simulink model "narx"  (R2019a)
settings: Solver=VariableStepAuto  StartTime=0.0  StopTime=10.0  RelTol=1e-3
libraries: neural x208
(part 2 of 4)

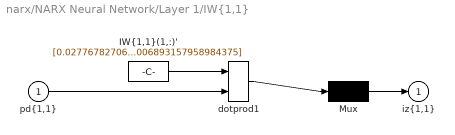
== system narx/NARX Neural Network/Layer 1/IW{1,1} ==
  "pd{1,1}" : Inport  PortDimensions=400  SampleTime=0.1
      mask Display: e = 0.06;c1 = [120 230 180]/255;c2 = ([120 230 180]+0)/(256+128);c3 = ([120 230 180]+128)/(256+128);patch([0 1 1 0],[0 0 1 1],c1);patch([0 1 1 1-e 1-e 0+e],[0 0 1 1-e 0+e 0+e],c2);patch([0 0 1 1-e 0+e 0+e],[0 1 1 1-e 1-e 0+e],c3);plot([0 1 1 0 0],[0 0 1 1 0]);
  "IW{1,1}(1,:)'" : Constant  Value=[0.0277678270648271420528718778086840757168829441070556640625;-0.072495516445331864563428325709537602961063385009765625;0.0729014756815358488939438075249199755489826202392578125;-0.07750431119418264847009680806877440772950649261474609375;0.08403681875376804721877732617940637283027172088623046875;0.034610402156992348121633540358743630349636077880859375;0.062177287459774917277588457409365219064056873321533203125;-0.055599584925755320130580372506301500834524631500244140625;0.03306038363780137989689222877132124267518520355224609375;0.059884523458899295567103848725309944711625576019287109375;-0.045214944417939294252217763414591900072991847991943359375;-0.06297951265383126828734106084084487520158290863037109375;-0.07549611905665236377682703050595591776072978973388671875;0.0244025606892776560086222303880276740528643131256103515625;-0.07090652620408342821090030838604434393346309661865234375;0.046678136882927552531175052763501298613846302032470703125;0.01041356304968433198199218026047674356959760189056396484375;-0.0682147965948884105191751814345479942858219146728515625;0.0395052435226136144930109139750129543244838714599609375;-0.01285278232501787902541945385337385232560336589813232421875;0.0297225523606888426819683246549175237305462360382080078125;0.052786377986352495117472471974906511604785919189453125;0.06689768777292716406268624496078700758516788482666015625;0.029275876104348765027740597588490345515310764312744140625;0.056569434444663994898672143563089775852859020233154296875;0.0801803794504956091060421385918743908405303955078125;0.04308993957098707083819277841030270792543888092041015625;0.01449172193578054414209166367299985722638666629791259765625;0.07754270635757322394088220107732922770082950592041015625;-0.04770856845629760367710758828252437524497509002685546875;-0.049209625536573896320557963690589531324803829193115234375;0.0831284199689841518665645025976118631660938262939453125;0.0035056066225432809015105650729537956067360937595367431640625;-0.0437420353957994889615434885854483582079410552978515625;-0.018606367207281183928646584035959676839411258697509765625;-0.04804876946083826150246665065424167551100254058837890625;-0.03351981478313360851561952813426614739000797271728515625;0.032643606251778249649486696171152289025485515594482421875;0.021534071288703326985114472336135804653167724609375;-0.06660372496869400305019581765009206719696521759033203125;-0.035615956814750070191788466900106868706643581390380859375;0.0179231172393173980583735982463622349314391613006591796875;0.06328180682564453485294819756745710037648677825927734375;0.054315872080360309837043786274080048315227031707763671875;-0.02052611847061401595393448360482580028474330902099609375;-0.0021784938142405513815391682186373145668767392635345458984375;0.0478869794394115866342787057874375022947788238525390625;-0.047002427956548124832192314670464838854968547821044921875;-0.0578385735760633679092279635369777679443359375;-0.042262951181773596165403006352789816446602344512939453125;0.08173333373884129893216510254205786623060703277587890625;0.007633612464141942451079092535337622393853962421417236328125;0.0286695925062813126993344070569946779869496822357177734375;0.0301009651872837340202959666157767060212790966033935546875;0.0200074381308329267425971664806638727895915508270263671875;-0.0728720042760638564427466690176515839993953704833984375;-0.005924178409521227255118969168279363657347857952117919921875;-0.02458613042365609402395421057008206844329833984375;0.018579335229139327945180326651097857393324375152587890625;0.0197572222726313286023103188426830456592142581939697265625;-0.03253055515353310556125876473743119277060031890869140625;0.058288896225512872029117517058693920262157917022705078125;-0.054834929476499406908462930232417420484125614166259765625;-0.083249590273886397984171026109834201633930206298828125;-0.04734203805234958595260508218416362069547176361083984375;0.006637613387688349846083024630161162349395453929901123046875 ...(+20044 chars)]
      mask Display: e = 0.06;c1 = [120 150 230]/255;c2 = ([120 150 230]+0)/383;c3 = ([120 150 230]+128)/383;patch([0 1 1 0],[0 0 1 1],c1);patch([0 1 1 1-e 1-e 0+e],[0 0 1 1-e 0+e 0+e],c2);patch([0 0 1 1-e 0+e 0+e],[0 1 1 1-e 1-e 0+e],c3);plot([0 1 1 0 0],[0 0 1 1 0]);disp('Weights');
  Mux : Mux  Inputs=1
      mask Display: e = 0.06;c1 = [120 150 230]/255;c2 = ([120 150 230]+0)/383;c3 = ([120 150 230]+128)/383;patch([0 1 1 0],[0 0 1 1],c1);patch([0 1 1 1-e 1-e 0+e],[0 0 1 1-e 0+e 0+e],c2);patch([0 0 1 1-e 0+e 0+e],[0 1 1 1-e 1-e 0+e],c3);plot([0 1 1 0 0],[0 0 1 1 0]);disp('Mux');
  dotprod1 : neural/Weight Functions/dotprod
      settings: SourceProductName=MATLAB Runtime - Deep Learning Toolbox  SourceProductBaseCode=Missing
  "iz{1,1}" : Outport
      mask Display: e = 0.06;c1 = [120 230 180]/255;c2 = ([120 230 180]+0)/(256+128);c3 = ([120 230 180]+128)/(256+128);patch([0 1 1 0],[0 0 1 1],c1);patch([0 1 1 1-e 1-e 0+e],[0 0 1 1-e 0+e 0+e],c2);patch([0 0 1 1-e 0+e 0+e],[0 1 1 1-e 1-e 0+e],c3);plot([0 1 1 0 0],[0 0 1 1 0]);
  wires:
  "IW{1,1}(1,:)'"/1 -> dotprod1/1
  "pd{1,1}"/1 -> dotprod1/2
  dotprod1/1 -> Mux/1
  Mux/1 -> "iz{1,1}"/1
